simulink library "LanekeepingBlocks"  (Simulink 7.2)
settings: Solver=ode45  StartTime=0.0  StopTime=10.0  RelTol=1e-3
values from neighbouring files (symbols this model uses):
  Ts = 0.002    [DSC_Control_Analysis.m]    (also in DSC_Control_Analysis_Exp.m; DSC_Speed_Control_Analysis.m; EC_params_nissan.m; Ext_MPCPara.m = SSD.Ts)
undefined symbols (not defined in the file or in its folder): DenYaw, K_fullstate, NumYaw
settings Model: Creator=ddl  LastModifiedBy=ddl

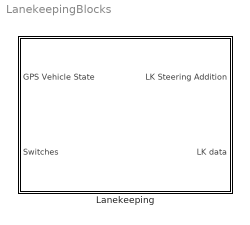
== system LanekeepingBlocks ==
  Lanekeeping : Subsystem

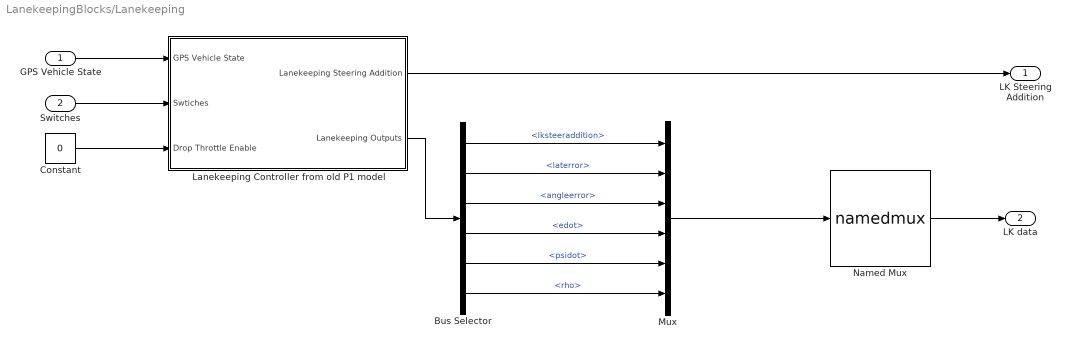
== system LanekeepingBlocks/Lanekeeping ==
  GPS Vehicle State : Inport
  Switches : Inport  Port=2
  Bus Selector : BusSelector  OutputSignals=lksteeraddition,laterror,angleerror,edot,psidot,rho
  Constant : Constant  Value=0  OutDataType=sfix(16)  OutScaling=2^0
  Lanekeeping Controller from old P1 model : Subsystem  mask{lkenable=on, disableondrop=off}
      mask prompts: lkenable "Enable Lanekeeping"; disableondrop "Disable Lanekeeping on Dropped Throttle"
      mask init:
      | p1_params;
      | lk_params_KT;
      | 
      | lkswitch = [gcs '/Lanekeeping Controller from old P1 model' '/Enable Lanekeeping'];
      | disableondropswitch = [gcs '/Lanekeeping Controller from old P1 model' '/Disable on Drop'];
      | set_param(lkswitch, 'value', '0');
      | set_param(disableondropswitch, 'value', '0');
      | 
      | if (lkenable == 1)
      |     set_param(lkswitch, 'value', '1');
      | end
      | 
      | if (disableondrop == 1)
      |     set_param(disableondropswitch, 'value', '1');
      | end
  Mux : Mux  Inputs=6
  Named Mux : S-Function  FunctionName=namedmux  Parameters=inputcount,inputsizes  EnableBusSupport=off  mask{fname=datadescLK}
      mask prompts: fname "Data description function name"
      mask help:
      | Combines input signals into a single output vector, according to a structure that provides the names and sizes of each signal.
      |
      | The parameter below should be set to the name of a function which returns a 1xN structure array, where N is the number of input signals.  The structure should contain fields "size" which specifies the width of the input signal, and "name" which specifies its name.
      mask init:
      | desc=eval(fname);
      | %if(class(desc)~='cell')
      | %	error('Incorrect description');
      | %end
      | inputcount=length(desc);
      | if((inputcount<1)|(inputcount>50))
      | 	error('Inappropriate number of inputs.');
      | end
      | 
      | inputsizes=[desc.size];
      | 
      | x=min(inputcount*ones(1,50),1:50);
      mask Display:
      | port_label('input',x(1),desc(x(1)).name);
      | port_label('input',x(2),desc(x(2)).name);
      | port_label('input',x(3),desc(x(3)).name);
      | port_label('input',x(4),desc(x(4)).name);
      | port_label('input',x(5),desc(x(5)).name);
      | port_label('input',x(6),desc(x(6)).name);
      | port_label('input',x(7),desc(x(7)).name);
      | port_label('input',x(8),desc(x(8)).name);
      | port_label('input',x(9),desc(x(9)).name);
      | port_label('input',x(10),desc(x(10)).name);
      | port_label('input',x(11),desc(x(11)).name);
      | port_label('input',x(12),desc(x(12)).name);
      | port_label('input',x(13),desc(x(13)).name);
      | port_label('input',x(14),desc(x(14)).name);
      | port_label('input',x(15),desc(x(15)).name);
      | port_label('input',x(16),desc(x(16)).name);
      | port_label('input',x(17),desc(x(17)).name);
      | port_label('input',x(18),desc(x(18)).name);
      | port_label('input',x(19),desc(x(19)).name);
      | port_label('input',x(20),desc(x(20)).name);
      | port_label('input',x(21),desc(x(21)).name);
      | port_label('input',x(22),desc(x(22)).name);
      | port_label('input',x(23),desc(x(23)).name);
      | port_label('input',x(24),desc(x(24)).name);
      | port_label('input',x(25),desc(x(25)).name);
      | port_label('input',x(26),desc(x(26)).name);
      | port_label('input',x(27),desc(x(27)).name);
      | port_label('input',x(28),desc(x(28)).name);
      | port_label('input',x(29),desc(x(29)).name);
      | port_label('input',x(30),desc(x(30)).name);
  LK Steering Addition : Outport
  LK data : Outport  Port=2
  wires:
  Bus Selector/6 -> Mux/6  "<rho>"
  Bus Selector/5 -> Mux/5  "<psidot>"
  Bus Selector/4 -> Mux/4  "<edot>"
  Bus Selector/3 -> Mux/3  "<angleerror>"
  Bus Selector/2 -> Mux/2  "<laterror>"
  Bus Selector/1 -> Mux/1  "<lksteeraddition>"
  Lanekeeping Controller from old P1 model/1(Lanekeeping Steering Addition) -> LK Steering Addition/1
  Switches/1 -> Lanekeeping Controller from old P1 model/2(Swtiches)
  GPS Vehicle State/1 -> Lanekeeping Controller from old P1 model/1(GPS Vehicle State)
  Mux/1 -> Named Mux/1
  Constant/1 -> Lanekeeping Controller from old P1 model/3(Drop Throttle Enable)
  Lanekeeping Controller from old P1 model/2(Lanekeeping Outputs) -> Bus Selector/1
  Named Mux/1 -> LK data/1

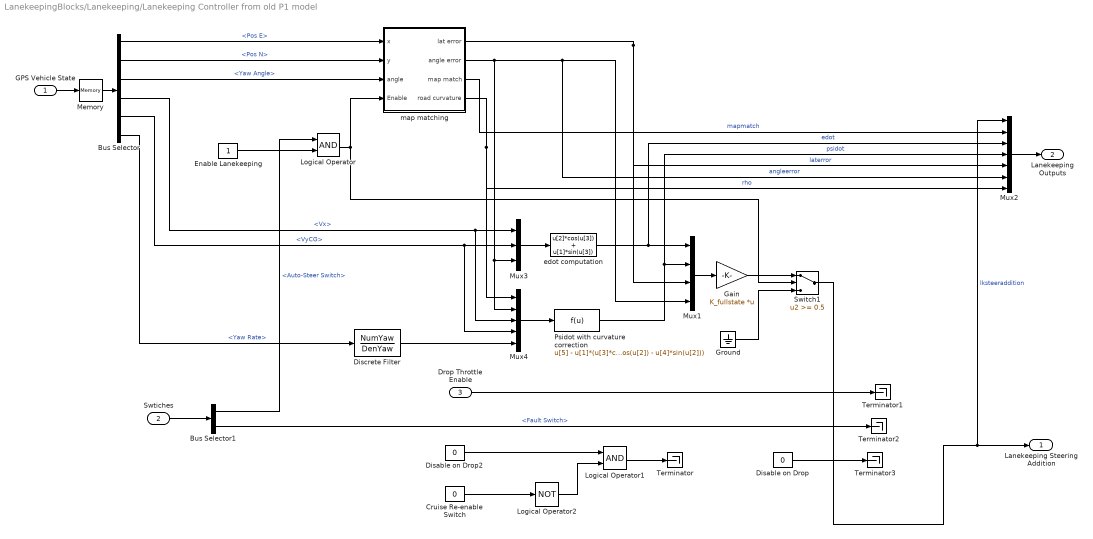
== system LanekeepingBlocks/Lanekeeping/Lanekeeping Controller from old P1 model ==
  GPS Vehicle State : Inport  OutDataType=sfix(16)  OutScaling=2^0
  Swtiches : Inport  Port=2  OutDataType=sfix(16)  OutScaling=2^0
  Drop Throttle Enable : Inport  Port=3  OutDataType=sfix(16)  OutScaling=2^0
  Bus Selector : BusSelector  OutputSignals=Pos E,Pos N,Yaw Angle,Vx,VyCG,Yaw Rate
  Bus Selector1 : BusSelector  OutputSignals=Auto-Steer Switch,Fault Switch
  Cruise Re-enable Switch : Constant  Value=0  OutDataType=sfix(16)  OutScaling=2^0
  Disable on Drop : Constant  Value=0  OutDataType=sfix(16)  OutScaling=2^0
  Disable on Drop2 : Constant  Value=0  OutDataType=sfix(16)  OutScaling=2^0
  Discrete Filter : DiscreteFilter  Numerator=NumYaw  Denominator=DenYaw  SampleTime=Ts
  Enable Lanekeeping : Constant  OutDataType=sfix(16)  OutScaling=2^0
  Gain : Gain  Gain=K_fullstate  Multiplication=Matrix(K*u)  ParameterDataType=sfix(16)  ParameterScaling=2^0  OutDataType=sfix(16)  OutScaling=2^0
  Ground : Ground
  Logical Operator : Logic  AllPortsSameDT=off  OutDataTypeMode=Specify via dialog  LogicDataType=float('double')  OutDataTypeStr=float('double')
  Logical Operator1 : Logic  AllPortsSameDT=off  OutDataTypeMode=Specify via dialog  LogicDataType=float('double')  OutDataTypeStr=float('double')
  Logical Operator2 : Logic  Operator=NOT  AllPortsSameDT=off  OutDataTypeMode=Specify via dialog  LogicDataType=float('double')  OutDataTypeStr=float('double')
  Memory : Memory
  Mux1 : Mux
  Mux2 : Mux  Inputs=7
  Mux3 : Mux  Inputs=3
  Mux4 : Mux  Inputs=5
  Psidot with curvature correction : Fcn  Expr=u[5] - u[1]*(u[3]*cos(u[2]) - u[4]*sin(u[2]))
  Switch1 : Switch  Threshold=0.5
  Terminator{,1..3} (4 alike) : Terminator
  edot computation : Fcn  Expr=u[2]*cos(u[3]) + u[1]*sin(u[3])
  map matching : Subsystem
  Lanekeeping Steering Addition : Outport  OutDataType=sfix(16)  OutScaling=2^0
  Lanekeeping Outputs : Outport  Port=2  OutDataType=sfix(16)  OutScaling=2^0
  wires:
  map matching/2(angle error) -> Mux3/3, Mux4/2, Mux1/4, Mux2/6  "angleerror"
  map matching/1(lat error) -> Mux1/3, Mux2/5  "laterror"
  map matching/3(map match) -> Mux2/2  "mapmatch"
  Mux2/1 -> Lanekeeping Outputs/1
  Bus Selector/3 -> map matching/3(angle)  "<Yaw Angle>"
  Bus Selector/2 -> map matching/2(y)  "<Pos N>"
  Bus Selector/1 -> map matching/1(x)  "<Pos E>"
  Logical Operator/1 -> Switch1/2, map matching/4(Enable)
  Enable Lanekeeping/1 -> Logical Operator/2
  Bus Selector/4 -> Mux3/1, Mux4/3  "<Vx>"
  Bus Selector/5 -> Mux3/2, Mux4/4  "<VyCG>"
  Mux1/1 -> Gain/1
  Mux3/1 -> edot computation/1
  edot computation/1 -> Mux1/1, Mux2/3  "edot"
  Gain/1 -> Switch1/1
  Ground/1 -> Switch1/3
  Bus Selector/6 -> Discrete Filter/1  "<Yaw Rate>"
  Drop Throttle Enable/1 -> Terminator1/1
  Swtiches/1 -> Bus Selector1/1
  Bus Selector1/1 -> Logical Operator/1  "<Auto-Steer Switch>"
  Bus Selector1/2 -> Terminator2/1  "<Fault Switch>"
  Switch1/1 -> Lanekeeping Steering Addition/1, Mux2/1  "lksteeraddition"
  Cruise Re-enable Switch/1 -> Logical Operator2/1
  Logical Operator2/1 -> Logical Operator1/2
  Disable on Drop2/1 -> Logical Operator1/1
  Memory/1 -> Bus Selector/1
  GPS Vehicle State/1 -> Memory/1
  map matching/4(road curvature) -> Mux4/1, Mux2/7  "rho"
  Discrete Filter/1 -> Mux4/5
  Mux4/1 -> Psidot with curvature correction/1
  Psidot with curvature correction/1 -> Mux1/2, Mux2/4  "psidot"
  Disable on Drop/1 -> Terminator3/1
  Logical Operator1/1 -> Terminator/1

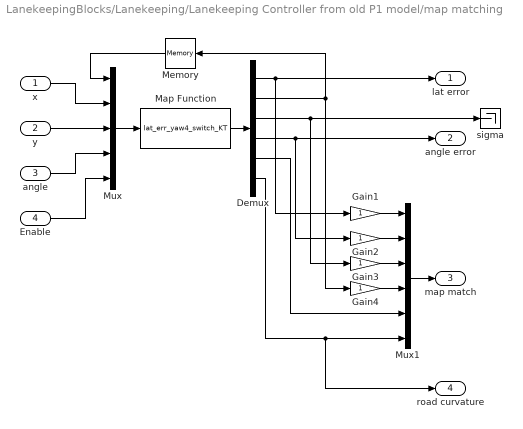
== system LanekeepingBlocks/Lanekeeping/Lanekeeping Controller from old P1 model/map matching ==
  x : Inport  OutDataType=sfix(16)  OutScaling=2^0
  y : Inport  Port=2  OutDataType=sfix(16)  OutScaling=2^0
  angle : Inport  Port=3  OutDataType=sfix(16)  OutScaling=2^0
  Enable : Inport  Port=4  OutDataType=sfix(16)  OutScaling=2^0
  Demux : Demux  Outputs=6
  Gain{1..4} (4 alike) : Gain  ParameterDataType=sfix(16)  ParameterScaling=2^0  OutDataType=sfix(16)  OutScaling=2^0  SaturateOnIntegerOverflow=on  OutDataTypeStr=Inherit: Same as input  ParamDataTypeStr=Inherit: Same as input
  Map Function : S-Function  FunctionName=lat_err_yaw4_switch_KT  EnableBusSupport=off
  Memory : Memory  Orientation=left
  Mux : Mux  Inputs=5
  Mux1 : Mux  Inputs=6
  sigma : Terminator
  lat error : Outport  OutDataType=sfix(16)  OutScaling=2^0
  angle error : Outport  Port=2  OutDataType=sfix(16)  OutScaling=2^0
  map match : Outport  Port=3  OutDataType=sfix(16)  OutScaling=2^0
  road curvature : Outport  Port=4  OutDataType=sfix(16)  OutScaling=2^0
  wires:
  Mux/1 -> Map Function/1
  Demux/1 -> lat error/1, Gain1/1
  Memory/1 -> Mux/1
  Demux/2 -> Gain4/1, Memory/1
  y/1 -> Mux/3
  Demux/3 -> Gain3/1, sigma/1
  Demux/4 -> angle error/1, Gain2/1
  Mux1/1 -> map match/1
  Map Function/1 -> Demux/1
  Gain1/1 -> Mux1/1
  Gain2/1 -> Mux1/2
  Gain3/1 -> Mux1/3
  Gain4/1 -> Mux1/4
  Enable/1 -> Mux/5
  x/1 -> Mux/2
  angle/1 -> Mux/4
  Demux/5 -> Mux1/5
  Demux/6 -> Mux1/6, road curvature/1
